simulink model "prelab"  (R2025b)
settings: Solver=VariableStepAuto  StartTime=0.0  StopTime=10.0  RelTol=1e-3
settings Model: Creator=eonuf  LastModifiedBy=eonuf

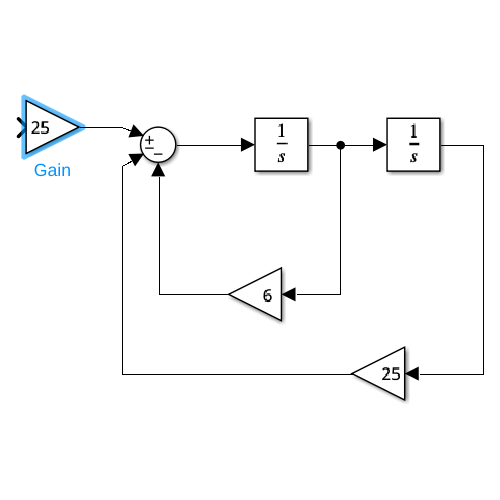
[thumbnail: Simulink's stored preview of the top-level diagram]
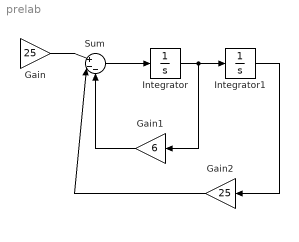
== system prelab ==
  Gain : Gain  Gain=25
  Gain1 : Gain  Gain=6
  Gain2 : Gain  Gain=25
  Integrator : Integrator
  Integrator1 : Integrator
  Sum : Sum  Inputs=|+--
  wires:
  Gain/1 -> Sum/1
  Integrator/1 -> Gain1/1, Integrator1/1
  Sum/1 -> Integrator/1
  Integrator1/1 -> Gain2/1
  Gain1/1 -> Sum/3
  Gain2/1 -> Sum/2
